simulink model "SerialCommunicationsTest"  (R2022b)
settings: Solver=FixedStepAuto  StartTime=0.0  StopTime=10.0  FixedStep=1e-3  RelTol=1e-3  EnableMultiTasking=on
libraries: frdmk64flib x5
settings Model: ExtModeTrigDuration=5  Creator=Admin  LastModifiedBy=Admin
settings OptimizationCC: EnhancedBackFolding=on  PassReuseOutputArgsAs=Individual arguments  ZeroExternalMemoryAtStartup=off  ZeroInternalMemoryAtStartup=off  MaxStackSize=64  OptimizeBlockOrder=speed  DifferentSizesBufferReuse=on  OptimizationCustomize=off  EfficientTunableParamExpr=on
settings DebuggingCC: ParameterTunabilityLossMsg=error
settings HardwareCC: ProdBitPerPointer=32  ProdBitPerSizeT=32  ProdBitPerPtrDiffT=32  ProdLargestAtomicInteger=Long  ProdLargestAtomicFloat=Double  ProdWordSize=32  ProdHWDeviceType=ARM Compatible->ARM Cortex
settings SFSimCC: MATLABDynamicMemAlloc=off
settings RTWCC: Description=Embedded Coder  SystemTargetFile=ert.tlc  HardwareBoard=NXP FRDM-K64F  TLCOptions="-aInlineSetEventsForThisBaseRateFcn=TLC_FALSE -aSuppressMultiTaskScheduler=TLC_FALSE  -aRateBasedStepFcn=0"  TemplateMakefile=ert_default_tmf  Toolchain=GNU Tools for ARM Embedded Processors
settings CodeAppCC: ForceParamTrailComments=on  IgnoreCustomStorageClasses=off  OperatorAnnotations=on  SimulinkDataObjDesc=on  SFDataObjDesc=on  InsertBlockDesc=on
settings ERTTargetCC: ExtModeTransport=4  ExtModeMexFile=sendToCommService

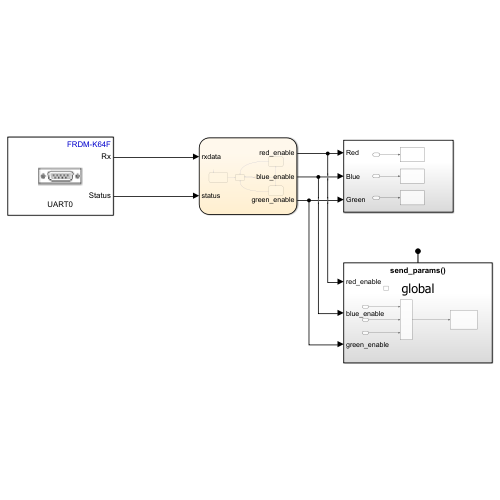
[thumbnail: Simulink's stored preview of the top-level diagram]
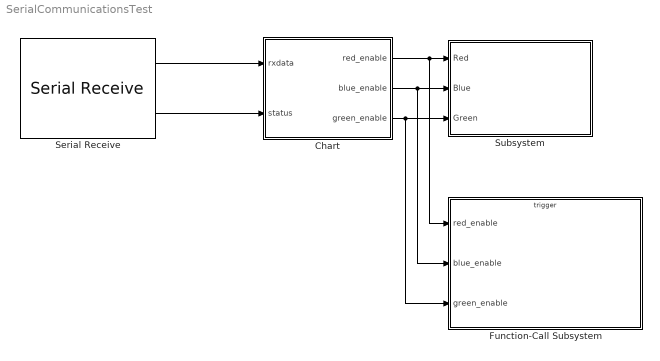
== system SerialCommunicationsTest ==
  Chart : Stateflow chart  TreatAsAtomicUnit=on
  Function-Call Subsystem : Subsystem  TreatAsAtomicUnit=on
  Serial Receive : frdmk64flib/Serial Receive  SCIModule=0  Baudrate=uint32(9600)  Parity=None  StopBits=1  HardwareFlowControl=None  ByteOrder=LittleEndian  DataType=uint8  DataLength=5  BlockingMode=off  OutputStatus=on  SampleTime=0.1
  Subsystem : Subsystem
  wires:
  Chart/3(green_enable) -> Function-Call Subsystem/3(green_enable), Subsystem/3(Green)
  Serial Receive/1 -> Chart/1(rxdata)
  Chart/2(blue_enable) -> Function-Call Subsystem/2(blue_enable), Subsystem/2(Blue)
  Chart/1(red_enable) -> Function-Call Subsystem/1(red_enable), Subsystem/1(Red)
  Serial Receive/2 -> Chart/2(status)

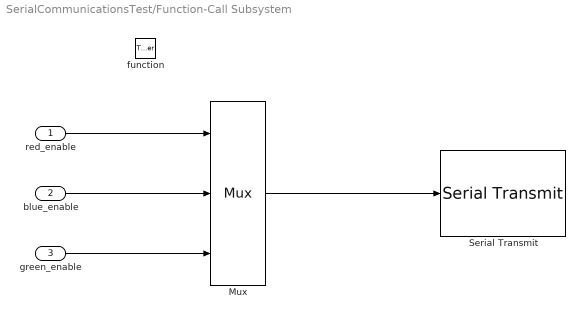
== system SerialCommunicationsTest/Function-Call Subsystem ==
  red_enable : Inport
  blue_enable : Inport  Port=2
  green_enable : Inport  Port=3
  function : TriggerPort  TriggerType=function-call  IsSimulinkFunction=on  FunctionName=send_params  VariantControl=(inherit)
  Mux : Mux  Inputs=3
      settings: DisplayOption=signals
  Serial Transmit : frdmk64flib/Serial Transmit  SCIModule=0  Baudrate=uint32(9600)  Parity=None  StopBits=1  HardwareFlowControl=None  ByteOrder=LittleEndian  BlockingMode=on  OutputStatus=off
  wires:
  red_enable/1 -> Mux/1
  blue_enable/1 -> Mux/2
  green_enable/1 -> Mux/3
  Mux/1 -> Serial Transmit/1

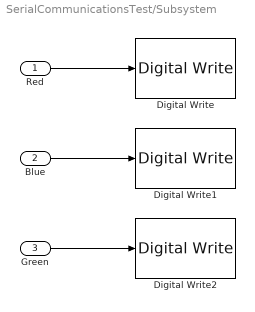
== system SerialCommunicationsTest/Subsystem ==
  Red : Inport
  Blue : Inport  Port=2
  Green : Inport  Port=3
  Digital Write : frdmk64flib/Digital Write  Whichpin=RED_LED
  Digital Write1 : frdmk64flib/Digital Write  Whichpin=BLUE_LED
  Digital Write2 : frdmk64flib/Digital Write  Whichpin=GREEN_LED
  wires:
  Green/1 -> Digital Write2/1
  Blue/1 -> Digital Write1/1
  Red/1 -> Digital Write/1

== stateflow chart SerialCommunicationsTest/Chart ==
  state Set_Params
    entry:
    red_enable = rxdata(3);
    blue_enable = rxdata(4);
    green_enable = rxdata(5);
  state Initial_State
    entry:
    %Setting initial parameters
    red_enable = 0;
    blue_enable = 0;
    green_enable = 0;
  state Standby
    %Waiting
  state Echo_params
    entry:
    send_params();
  Set_Params -> Standby
  (junction 4) -> Set_Params [order 2] : [rxdata(2)==55]
  (default) -> Initial_State
  (junction 8) -> Standby [order 2]
  Standby -> (junction 8) : [status == 0]
  (junction 8) -> (junction 4) [order 1] : [rxdata(1) == 16]
  Initial_State -> Standby
  (junction 4) -> Echo_params [order 1] : [rxdata(2)==22]
  Echo_params -> Standby
  data: red_enable output uint8; rxdata input; status input; blue_enable output uint8; green_enable output uint8
